simulink model "ModbusTCP_Test"  (R2023a)
settings: Solver=FixedStepAuto  StartTime=0.0  StopTime=10.0  FixedStep=1  RelTol=1e-3
libraries: realtime_pacer_lib x1
settings Model: Creator=Christian  LastModifiedBy=Christian

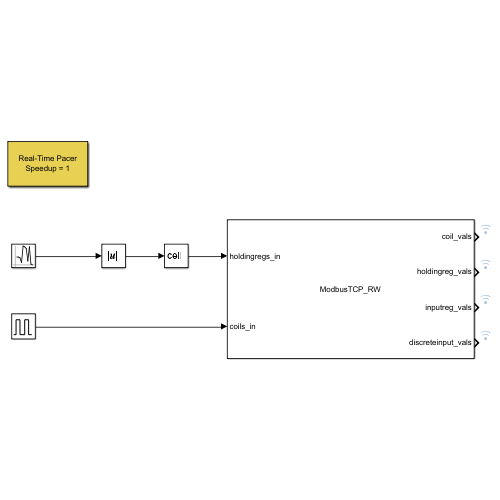
[thumbnail: Simulink's stored preview of the top-level diagram]
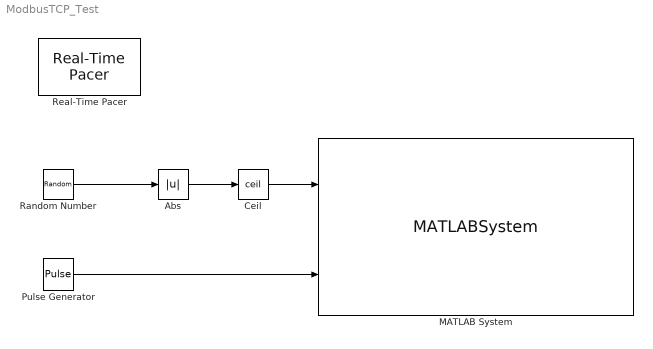
== system ModbusTCP_Test ==
  Abs : Abs  SaturateOnIntegerOverflow=off
  Ceil : Rounding  Operator=ceil
  MATLAB System : MATLABSystem  System=ModbusTCP_RW  address=127.0.0.1  port=5020  sampling_time=1  coils_to_read=10  coils_read_start=1  hr_to_read=10  hr_read_start=1  di_to_read=10  di_read_start=1  ir_to_read=10  ir_read_start=1  coils_write_start=1  hr_write_start=1  SimulateUsing=Interpreted execution
      mask Type: ModbusTCP_RW
      mask Display:
      | disp('ModbusTCP_RW');
      | port_label('input',1,'holdingregs_in');
      | port_label('input',2,'coils_in');
      | port_label('output',1,'coil_vals');
      | port_label('output',2,'holdingreg_vals');
      | port_label('output',3,'inputreg_vals');
      | port_label('output',4,'discreteinput_vals');
  Pulse Generator : DiscretePulseGenerator  PulseType=Time based  PulseWidth=50
  Random Number : RandomNumber  Variance=ones(5,1)  SampleTime=1
  Real-Time Pacer : realtime_pacer_lib/Real-Time Pacer  simTimePerRealTime=1
      settings: SourceProductName=Real-Time Pacer
  wires:
  Random Number/1 -> Abs/1
  Abs/1 -> Ceil/1
  Ceil/1 -> MATLAB System/1
  Pulse Generator/1 -> MATLAB System/2
